simulink model "TPS"  (R2022b)
settings: Solver=FixedStepDiscrete  StartTime=0.0  StopTime=10.0  FixedStep=0.1  RelTol=1e-3
settings Model: Creator=ahmed  LastModifiedBy=ahmed

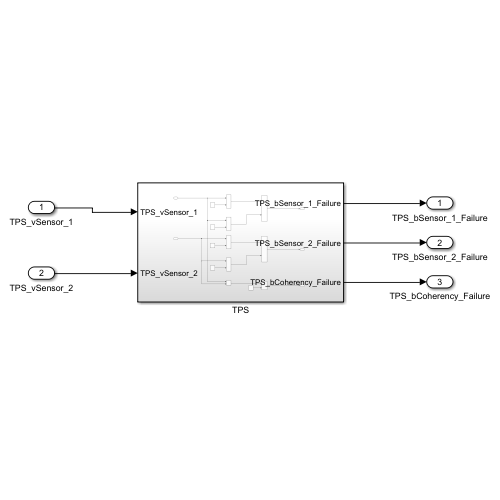
[thumbnail: Simulink's stored preview of the top-level diagram]
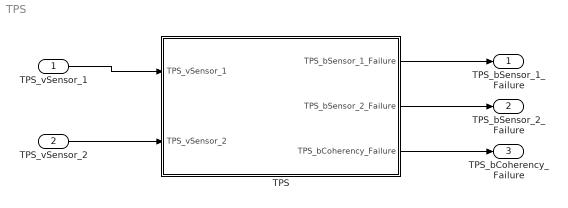
== system TPS ==
  TPS_vSensor_1 : Inport  OutDataTypeStr=single
  TPS_vSensor_2 : Inport  Port=2  OutDataTypeStr=single
  TPS : Subsystem
  TPS_bSensor_1_Failure : Outport  OutDataTypeStr=boolean
  TPS_bSensor_2_Failure : Outport  Port=2  OutDataTypeStr=boolean
  TPS_bCoherency_Failure : Outport  Port=3  OutDataTypeStr=boolean
  wires:
  TPS_vSensor_1/1 -> TPS/1(TPS_vSensor_1)
  TPS_vSensor_2/1 -> TPS/2(TPS_vSensor_2)
  TPS/1(TPS_bSensor_1_Failure) -> TPS_bSensor_1_Failure/1
  TPS/2(TPS_bSensor_2_Failure) -> TPS_bSensor_2_Failure/1
  TPS/3(TPS_bCoherency_Failure) -> TPS_bCoherency_Failure/1

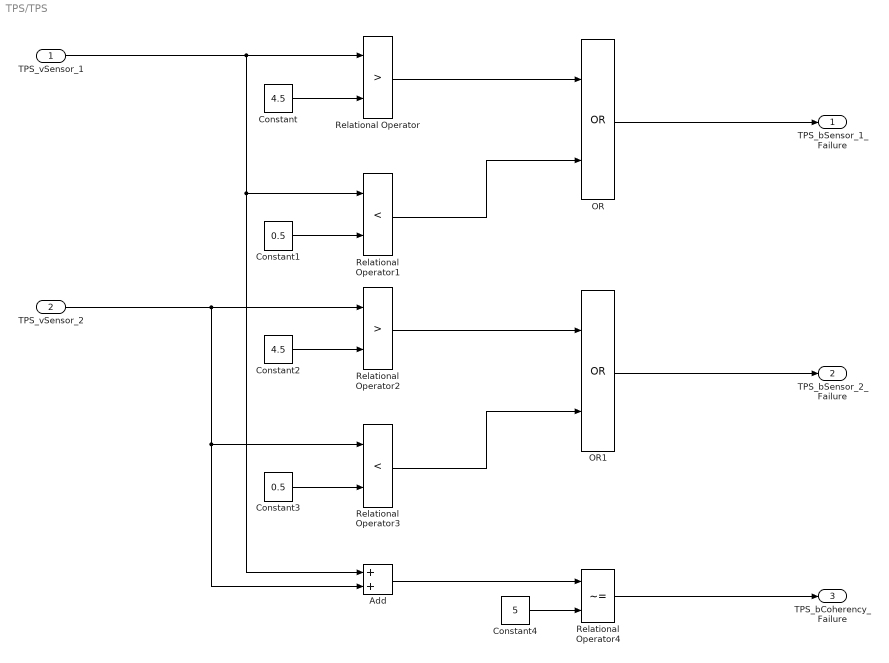
== system TPS/TPS ==
  TPS_vSensor_1 : Inport  OutDataTypeStr=single
  TPS_vSensor_2 : Inport  Port=2  OutDataTypeStr=single
  Add : Sum
  Constant : Constant  Value=4.5  OutDataTypeStr=single
  Constant1 : Constant  Value=0.5  OutDataTypeStr=single
  Constant2 : Constant  Value=4.5  OutDataTypeStr=single
  Constant3 : Constant  Value=0.5  OutDataTypeStr=single
  Constant4 : Constant  Value=5
  OR : Logic  Operator=OR  AllPortsSameDT=off  OutDataTypeStr=boolean
  OR1 : Logic  Operator=OR  AllPortsSameDT=off  OutDataTypeStr=boolean
  Relational Operator : RelationalOperator  Operator=>  OutDataTypeStr=boolean  RndMeth=Simplest  InputSameDT=off
  Relational Operator1 : RelationalOperator  Operator=<  OutDataTypeStr=boolean  RndMeth=Simplest  InputSameDT=off
  Relational Operator2 : RelationalOperator  Operator=>  OutDataTypeStr=boolean  RndMeth=Simplest  InputSameDT=off
  Relational Operator3 : RelationalOperator  Operator=<  OutDataTypeStr=boolean  RndMeth=Simplest  InputSameDT=off
  Relational Operator4 : RelationalOperator  Operator=~=  OutDataTypeStr=boolean  RndMeth=Simplest  InputSameDT=off
  TPS_bSensor_1_Failure : Outport  OutDataTypeStr=boolean
  TPS_bSensor_2_Failure : Outport  Port=2  OutDataTypeStr=boolean
  TPS_bCoherency_Failure : Outport  Port=3  OutDataTypeStr=boolean
  wires:
  TPS_vSensor_2/1 -> Relational Operator2/1, Relational Operator3/1, Add/2
  Constant/1 -> Relational Operator/2
  Add/1 -> Relational Operator4/1
  Constant4/1 -> Relational Operator4/2
  Constant1/1 -> Relational Operator1/2
  OR1/1 -> TPS_bSensor_2_Failure/1
  OR/1 -> TPS_bSensor_1_Failure/1
  TPS_vSensor_1/1 -> Relational Operator/1, Relational Operator1/1, Add/1
  Relational Operator2/1 -> OR1/1
  Relational Operator3/1 -> OR1/2
  Relational Operator1/1 -> OR/2
  Constant3/1 -> Relational Operator3/2
  Constant2/1 -> Relational Operator2/2
  Relational Operator4/1 -> TPS_bCoherency_Failure/1
  Relational Operator/1 -> OR/1
